simulink model "project_model"  (R2024b)
settings: Solver=VariableStepAuto  StartTime=0.0  StopTime=120  FixedStep=0.01  RelTol=1e-3
settings Model: PacingRate=0.999000  Creator=Megha Shah  LastModifiedBy=Megha Shah

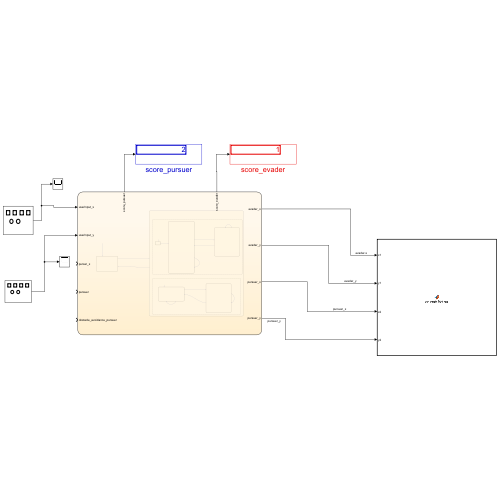
[thumbnail: Simulink's stored preview of the top-level diagram]
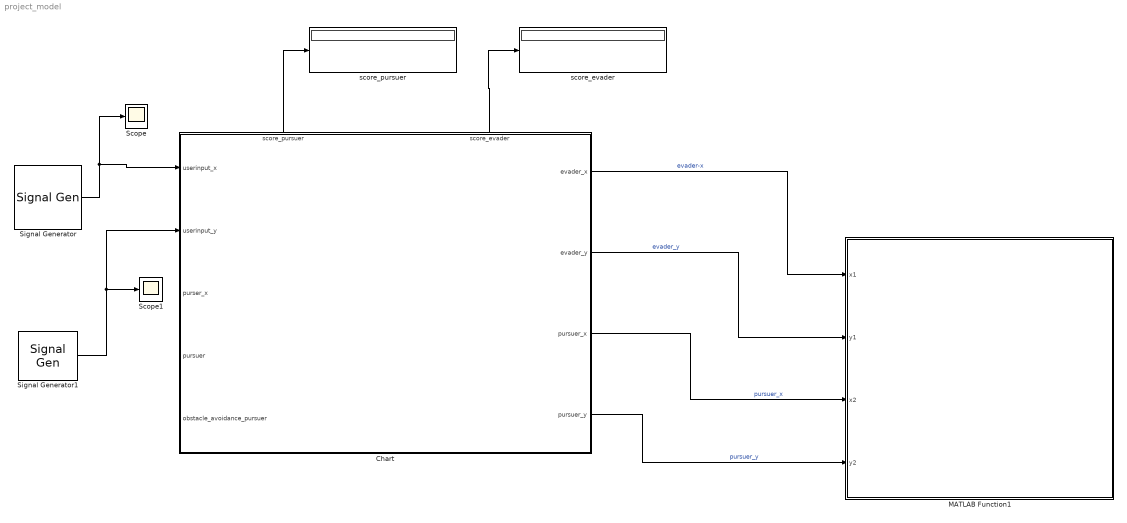
== system project_model ==
  Chart : Stateflow chart  TreatAsAtomicUnit=on
      settings: PortSchema="{\"entries\":[{\"content\":{\"sides\":[{\"content\":{\"connectorIds\":[\"In1\",\"In2\",\"In3\",\"In4\",\"In5\"]},\"type\":\"ConnectorPlacement.EquallySpacedRectSide\",\"uuid\":\"86b65d3c-6252-4204-be57-bca09b6cebb3\"},{\"content\":{\"connectorIds\":[\"Out3\",\"Out4\",\"Out5\",\"Out6\"],\"side\":\"RIGHT\"},\"type\":\"ConnectorPlacement.EquallySpacedRectSide\",\"uuid\":\"18a5d582-5651-41a9-b7b4-93b704f5850a\"},{\"content\":{\"connectorIds\":[\"Out1\",\"Out2\"],\"side\":\"TOP\"},\"type\":\"ConnectorPlacement.EquallySpacedRectSide\",\"uuid\":\"c8dfdba2-f5a5-4d66-8be7-61a2da2d2f4b\"}]},\"type\":\"ConnectorPlacement.EquallySpacedConnector\",\"uuid\":\"89cad2b9-92e4-438e-ad5e-0bc8c43f4802\"}],\"packageUris\":[\"http://schema.mathworks.com/mf0/Connector/R2020b\"],\"version\":\"1.0\"}"
  MATLAB Function1 : MATLAB Function  TreatAsAtomicUnit=on
  Scope : Scope
  Scope1 : Scope
  Signal Generator : SignalGenerator  WaveForm=random  Amplitude=3  Frequency=0.5
  Signal Generator1 : SignalGenerator  WaveForm=random  Amplitude=3
  score_evader : Display
  score_pursuer : Display
  wires:
  Chart/1(score_pursuer) -> score_pursuer/1
  Chart/2(score_evader) -> score_evader/1
  Chart/3(evader_x) -> MATLAB Function1/1(x1)  "evader-x"
  Chart/4(evader_y) -> MATLAB Function1/2(y1)  "evader_y"
  Chart/5(pursuer_x) -> MATLAB Function1/3(x2)  "pursuer_x"
  Chart/6(pursuer_y) -> MATLAB Function1/4(y2)  "pursuer_y"
  Signal Generator/1 -> Scope/1, Chart/1(userinput_x)
  Signal Generator1/1 -> Scope1/1, Chart/2(userinput_y)

== matlab function project_model/MATLAB Function1 ==
  data: x1 input; y1 input; x2 input; y2 input
function animateMotion(x1, y1, x2, y2)
    % Define a persistent figure and plot handles to avoid recreating them
    persistent h1 h2 fig;

    % Initialize the figure and plots if they don't exist
    if isempty(fig) 
        fig = figure; % Create a new figure
        hold on; % Allow multiple plots in the same figure
        h1 = plot(0, 0, 'ro', 'MarkerSize', 8, 'MarkerFaceColor', 'r'); % evader
        h2 = plot(0, 0, 'bo', 'MarkerSize', 8, 'MarkerFaceColor', 'b'); % pursuer

         % Plot the dotted square lines
        xSquare = [2, 8, 8, 2, 2];
        ySquare = [2, 2, 8, 8, 2];
        squareLines = plot(xSquare, ySquare, 'k--', 'LineWidth', 1); % Dotted square lines

        grid on;
        xlim([0 10]); ylim([0 10]); % Adjust axes as needed
        xlabel('X'); ylabel('Y');
        title('2D Motion Animation');
        hold off;
        legend('evader','pursuer','Location','northeastoutside');
    end

    % Update the positions of the two balls
    set(h1, 'XData', x1, 'YData', y1); % Update Ball 1
    set(h2, 'XData', x2, 'YData', y2); % Update Ball 2
    drawnow ; % Optimize figure updates
end

== stateflow chart project_model/Chart ==
  state Game1_ON
    en:
    obstacle_p=0;
    obstacle_e=0;
    caught=0;
    state Pursuer [parallel]
      settings: executionOrder=1
      state Tracking
        max_vel = 1;
        range_x=evader_x-pursuer_x;
        range_y=evader_y-pursuer_y;
        caught_dist = 1;
        if abs(range_x)<caught_dist && abs( range_y)<caught_dist
        caught =1;
        end
        yxratio = abs(range_y)/abs(range_x);
        if yxratio>max_vel
        if range_x>=0 && range_y>=0
        pursuer_x=pursuer_x+(1/yxratio)*max_vel;
        pursuer_y=pursuer_y+max_vel;
        elseif range_x<0 && range_y>=0
        pursuer_x=pursuer_x-(1/yxratio)*max_vel;
        pursuer_y=pursuer_y+max_vel;
        elseif range_x<0 && range_y<0
        pursuer_x=pursuer_x-(1/yxratio)*max_vel;
        pursuer_y=pursuer_y-max_vel;
        elseif range_x>=0 && range_y<0
        pursuer_x=pursuer_x+(1/yxratio)*max_vel;
        pursuer_y=pursuer_y-max_vel;
        else
        pursuer_x=pursuer_x;
        pursuer_y=pursuer_y
        end
        else
        if range_x>=0 && range_y>=0
        pursuer_x=pursuer_x+max_vel;
        pursuer_y=pursuer_y+yxratio*max_vel;
        elseif range_x<0 && range_y>=0
        pursuer_x=pursuer_x-max_vel;
        pursuer_y=pursuer_y+yxratio*max_vel;
        elseif range_x<0 && range_y<0
        pursuer_x=pursuer_x-max_vel;
        pursuer_y=pursuer_y-yxratio*max_vel;
        elseif range_x>=0 && range_y<0
        pursuer_x=pursuer_x+max_vel;
        pursuer_y=pursuer_y-yxratio*max_vel;
        else
        pursuer_x=pursuer_x;
        pursuer_y=pursuer_y
        end
        end
        if (pursuer_x>8 || pursuer_x<2 || pursuer_y>8 || pursuer_y<2)
        obstacle_p = 1;
        end
      state obstacle_avoidance_pursuer
        max_vel =1;
        if pursuer_y>8 && pursuer_x<8
        pursuer_x=pursuer_x+max_vel;
        pursuer_y=pursuer_y-max_vel;
        elseif pursuer_y<2 && pursuer_x<8
        pursuer_x=pursuer_x+max_vel;
        pursuer_y=pursuer_y+max_vel;
        elseif pursuer_y>8 && pursuer_x>2
        pursuer_x=pursuer_x-max_vel;
        pursuer_y=pursuer_y-max_vel;
        elseif pursuer_y<2 && pursuer_x<8
        pursuer_x=pursuer_x-max_vel;
        pursuer_y=pursuer_y+max_vel;
        elseif pursuer_x<2
        pursuer_x=pursuer_x+max_vel;
        pursuer_y=pursuer_y+max_vel;
        elseif pursuer_x>8
        pursuer_x=pursuer_x-max_vel;
        pursuer_y=pursuer_y-max_vel;
        end
        if (pursuer_x>8 || pursuer_x<2 || pursuer_y>8 || pursuer_y<2)
        obstacle_p =1
        else
        obstacle_p =0;
        end
      state timer_p
      obstacle_avoidance_pursuer -> obstacle_avoidance_pursuer [order 2] : [obstacle_p==1]
      (default) -> timer_p
      Tracking -> obstacle_avoidance_pursuer [order 1] : [obstacle_p==1]{pursuer_x,pursuer_y}
      timer_p -> Tracking : after(5,sec)
      obstacle_avoidance_pursuer -> Tracking [order 1] : [obstacle_p==0]{pursuer_x,pursuer_y}
      Tracking -> Tracking [order 2] : [obstacle_p==0]
    state Evader [parallel]
      settings: executionOrder=2
      state obstacle_avoidance_e
        max_vel =2;
        if evader_y>8 && evader_x<8
        evader_x=evader_x+max_vel;
        evader_y=evader_y-max_vel;
        elseif evader_y<2 && evader_x<8
        evader_x=evader_x+max_vel;
        evader_y=evader_y+max_vel;
        elseif evader_y>8 && evader_x>2
        evader_x=evader_x-max_vel;
        evader_y=evader_y-max_vel;
        elseif evader_y<2 && evader_x<8
        evader_x=evader_x-max_vel;
        evader_y=evader_y+max_vel;
        elseif evader_x<2
        evader_x=evader_x+max_vel;
        evader_y=evader_y+max_vel;
        elseif evader_x>8
        evader_x=evader_x-max_vel;
        evader_y=evader_y-max_vel;
        end
        if (evader_x>8 || evader_x<2 || evader_y>8 || evader_y<2)
        obstacle_e =1
        else
        obstacle_e =0;
        end
      state Human_control
        if (evader_x+userinput_x<9.5 && evader_x+userinput_x>0.5 )
        evader_x = evader_x+userinput_x;
        end
        if (evader_y+userinput_y<9.5 && evader_y+userinput_y>0.5)
        evader_y = evader_y+userinput_y;
        end
        if (evader_x>8 || evader_x<2 || evader_y>8 || evader_y<2)
        obstacle_e = 1;
        end
      (default) -> Human_control
      Human_control -> obstacle_avoidance_e [order 1] : [obstacle_e==1]{evader_x,evader_y}
      obstacle_avoidance_e -> obstacle_avoidance_e [order 2] : [obstacle_e==1]
      obstacle_avoidance_e -> Human_control [order 1] : [obstacle_e==0]{evader_x,evader_y}
      Human_control -> Human_control [order 2] : [obstacle_e==0]
  state Game_OFF
    if (caught==1)
    score_pursuer=score_pursuer+1
    elseif (caught==0)
    score_evader=score_evader+1
    end
    caught=-1;
  (default) -> Game_OFF : {caught=-1;
      | expired=0;
      | score_pursuer=0;
      | score_evader=0;
      | pursuer_x=3;
      | pursuer_y=3;
      | evader_x=7;
      | evader_y=7;}
  Game_OFF -> Game1_ON : after(5,sec)
  Game1_ON -> Game_OFF : [caught==1 || after(30,sec)]
  data: score_pursuer output; score_evader output; caught local; expired local; userinput_x input; userinput_y input; caught_dist local; max_vel local; purser_y local; range_x local; range_y local; timer local; yxratio local; evader_x output; evader_y output; pursuer_x output; pursuer_y output; prev_evader_x local; prev_evader_y local; obstacle_e local; obstacle_p local; purser_x input; pursuer input; obstacle_avoidance_pursuer input
